simulink model "gpc_siso_delay_1_sim"  (R2022a)
settings: Solver=VariableStepAuto  StartTime=0.0  StopTime=Tsim  RelTol=1e-3
values from neighbouring files (symbols this model uses):
  A = A'    [gpc_siso_delay_1.m]
  B = B'    [gpc_siso_delay_1.m]
  D = D'    [gpc_siso_delay_1.m]
  delta = 1    [gpc_siso_delay_1.m]
  H = H'    [gpc_siso_delay_1.m]
  KF = K*F    [gpc_siso_delay_1.m]
  KFFIR = KF*FFilter    [gpc_siso_delay_1.m]
  Kr = sum(K)    [gpc_siso_delay_1.m]
  Ld = ceil(L/Ts)    [gpc_siso_delay_1.m]
  Ts = 1    [gpc_siso_delay_1.m]
libraries: cstblocks x2
settings Model: Creator=aaron  LastModifiedBy=aaron

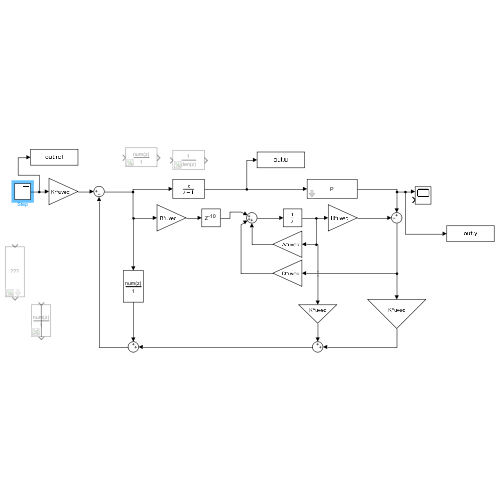
[thumbnail: Simulink's stored preview of the top-level diagram]
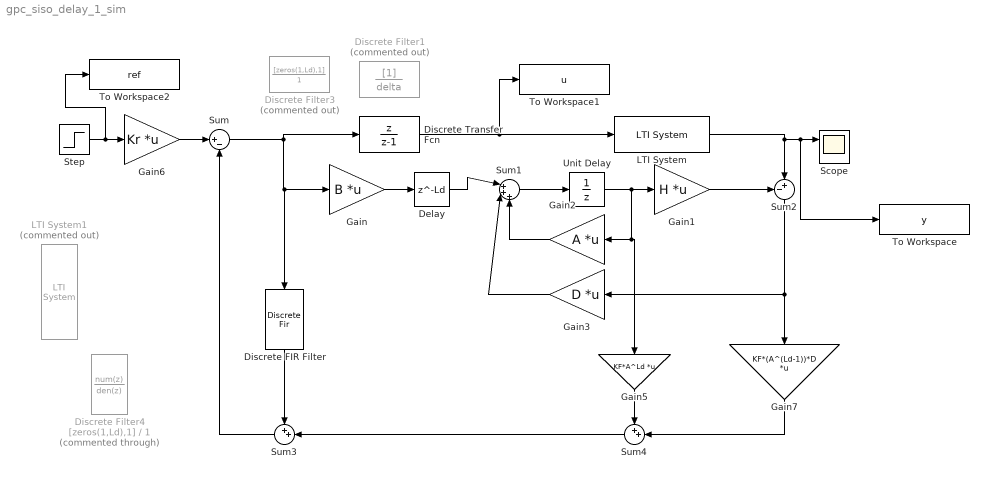
== system gpc_siso_delay_1_sim ==
  Delay : Delay  DelayLength=Ld  SampleTime=Ts
  Discrete Transfer Fcn : DiscreteTransferFcn  Numerator=[1 0]  Denominator=[1 -1]  SampleTime=Ts
  Discrete FIR Filter : DiscreteFir  Coefficients=KFFIR  SampleTime=Ts
  Discrete Filter1 : DiscreteFilter  Commented=on  Denominator=delta
  Discrete Filter3 : DiscreteFilter  Commented=on  Numerator=[zeros(1,Ld),1]  Denominator=1
  Discrete Filter4 : DiscreteFilter  Commented=through  Numerator=[zeros(1,Ld),1]  Denominator=1
  Gain : Gain  Gain=B  Multiplication=Matrix(K*u) (u vector)
  Gain1 : Gain  Gain=H  Multiplication=Matrix(K*u) (u vector)
  Gain2 : Gain  Gain=A  Multiplication=Matrix(K*u) (u vector)
  Gain3 : Gain  Gain=D  Multiplication=Matrix(K*u) (u vector)
  Gain5 : Gain  Gain=KF*A^Ld  Multiplication=Matrix(K*u) (u vector)
  Gain6 : Gain  Gain=Kr  Multiplication=Matrix(K*u) (u vector)
  Gain7 : Gain  Gain=KF*(A^(Ld-1))*D  Multiplication=Matrix(K*u) (u vector)
  LTI System : cstblocks/LTI System  sys=P  IC=[]
  LTI System1 : cstblocks/LTI System  Commented=on  sys=Ftil  IC=[]
  Scope : Scope  NumInputPorts=2
  Step : Step  Time=0  SampleTime=0
  Sum : Sum  Inputs=|+-
  Sum1 : Sum  Inputs=|+++
  Sum2 : Sum  Inputs=-+|
  Sum3 : Sum  Inputs=++|
  Sum4 : Sum  Inputs=++|
  To Workspace : ToWorkspace  VariableName=y  SampleTime=Ts
  To Workspace1 : ToWorkspace  VariableName=u  SampleTime=Ts
  To Workspace2 : ToWorkspace  VariableName=ref  SampleTime=Ts
  Unit Delay : UnitDelay  SampleTime=Ts  HasFrameUpgradeWarning=on
  wires:
  Gain6/1 -> Sum/1
  Step/1 -> To Workspace2/1, Gain6/1
  Sum1/1 -> Unit Delay/1
  Gain1/1 -> Sum2/1
  LTI System/1 -> To Workspace/1, Scope/1, Sum2/2
  Discrete Transfer Fcn/1 -> LTI System/1, To Workspace1/1
  Sum/1 -> Discrete Transfer Fcn/1, Gain/1, Discrete FIR Filter/1
  Unit Delay/1 -> Gain2/1, Gain5/1, Gain1/1
  Gain2/1 -> Sum1/3
  Sum2/1 -> Gain3/1, Gain7/1
  Gain3/1 -> Sum1/2
  Gain5/1 -> Sum4/1
  Gain7/1 -> Sum4/2
  Delay/1 -> Sum1/1
  Gain/1 -> Delay/1
  Sum4/1 -> Sum3/2
  Sum3/1 -> Sum/2
  Discrete FIR Filter/1 -> Sum3/1
